simulink model "ndtm_V2"  (R2018b)
settings: configuration reference "Physics" (kept outside this file)
model workspace (MAT data in the model file):
  x0_initialstates = [0 0 0 0 0 0]
undefined symbols (not defined in the file): F0z, h, INIT__initialvalues__Vehicle_InitialPitchRate_radps, INIT__initialvalues__Vehicle_InitialRollRate_radps, INIT__initialvalues__Vehicle_InitialVelocity_mps__1, INIT__initialvalues__Vehicle_InitialVelocity_mps__2, INIT__initialvalues__Vehicle_InitialVelocity_mps__3, INIT__initialvalues__Vehicle_InitialYawRate_radps, SUS__Antisway__c_AntiSwayTSpringFrRe_Nmprad__1, SUS__Antisway__c_AntiSwayTSpringFrRe_Nmprad__2, SUS__Antisway__phi_AntiSwayNeutralAngleFrRe_rad__1, SUS__Antisway__phi_AntiSwayNeutralAngleFrRe_rad__2, SUS__Antisway__r_AntiSwayArmRadiusFrRe_m__1, SUS__Antisway__r_AntiSwayArmRadiusFrRe_m__2, SUS__Compliance__Cz_DamperRateFrRe_Nspm__1, SUS__Compliance__Cz_DamperRateFrRe_Nspm__2, SUS__Compliance__cz_SpringRateFrRe_Npm__1, SUS__Compliance__cz_SpringRateFrRe_Npm__2, SUS__Compliance__F0z_SpringPreloadFrRe_N__1, SUS__Compliance__F0z_SpringPreloadFrRe_N__2, SUS__Compliance__h_InertialFrameOffset_COGtoAxle_m, SUS__Kinematics__k_CamberATSteerCenterF__1, SUS__Kinematics__k_CamberATSteerCenterF__2, SUS__Kinematics__k_CamberVSHeightFrRe__1, SUS__Kinematics__k_CamberVSHeightFrRe__2, SUS__Kinematics__k_CasterATSteerCenterF__1, SUS__Kinematics__k_CasterATSteerCenterF__2, SUS__Kinematics__k_CasterVSHeightFrRe__1, SUS__Kinematics__k_CasterVSHeightFrRe__2, SUS__Kinematics__k_RollSteerVSHeightFrRe_radpm__1, SUS__Kinematics__k_RollSteerVSHeightFrRe_radpm__2, SUS__Kinematics__nu0_ToeATSteerCenterFrRe_rad__1, SUS__Kinematics__nu0_ToeATSteerCenterFrRe_rad__2, tireFL__SCALING__LFZO, tireFR__SCALING__LFZO, tireRL__SCALING__LFZO, tireRR__SCALING__LFZO, VEH, VEH__Aerodynamics__beta_wind_end_rad, VEH__Aerodynamics__beta_wind_start_rad, VEH__Aerodynamics__beta_wind_step_rad, VEH__Aerodynamics__cl_LongitudinalLift, VEH__Aerodynamics__Cs_LatDragCoeff_end, VEH__Aerodynamics__Cs_LatDragCoeff_start, VEH__Aerodynamics__Cs_LatDragCoeff_step, VEH__Aerodynamics__Cym_DragYawMomentCoeff_end, VEH__Aerodynamics__Cym_DragYawMomentCoeff_start, VEH__Aerodynamics__Cym_DragYawMomentCoeff_step, VEH__Environment__a_Gravity_mps2, VEH__Tires__p_Tires_pa__1, VEH__Tires__p_Tires_pa__2, VEH__Tires__p_Tires_pa__3, VEH__Tires__p_Tires_pa__4, VEH__VehicleData__l_WheelbaseF_m, VEH__VehicleData__l_WheelbaseTotal_m, VEH__VehicleData__m_Vehicle_kg, VEH__VehicleData__w_GeomCenterlineToCOG_m, VEH__VehicleData__w_TrackF_m, VEH__VehicleData__w_TrackR_m
libraries: vehdynlibsuspension x7, vehdynlibtire x4, vehdynlibtire_TUM x4, autolibutils x2, sharedtransform x2, vehdynlibeom_TUM x1
(part 4 of 4)

== system ndtm_V2/Wheels and Tires/VDBS/Veh2Tire ==
  r : Inport
  Axle : Inport  Port=2
  Brake : Inport  Port=3
  VehVel : Inport  Port=4
  WheelSteer : Inport  Port=5
  WheelCamber : Inport  Port=6
  Demux4 : Demux
  Gain4 : Gain  Gain=[1;-1;1;-1]*0+1
  Mux1 : Mux
  Reshape3 : Reshape
  Reshape4 : Reshape
  Unary Minus : UnaryMinus
  Wheel Angles : Subsystem
  Wheel to Body Transform : Subsystem
  T : Outport  Unit=N*m
  P : Outport  Port=2  Unit=Pa
  psidot : Outport  Port=3  Unit=rad/s
  xdotAxle : Outport  Port=4  Unit=m/s
  ydotAxle : Outport  Port=5  Unit=m/s
  zdotAxle : Outport  Port=6  Unit=m/s
  wires:
  Demux4/1 -> Mux1/1
  Brake/1 -> Reshape3/1
  Demux4/4 -> Mux1/4
  Axle/1 -> Reshape4/1
  Wheel to Body Transform/1(xdotWheel) -> xdotAxle/1  "Vx"
  Demux4/2 -> Mux1/2
  Wheel to Body Transform/2(ydotWheel) -> ydotAxle/1  "Vy"
  WheelSteer/1 -> Wheel Angles/1(steer)
  Mux1/1 -> P/1
  r/1 -> Unary Minus/1
  Demux4/3 -> Mux1/3
  Reshape3/1 -> Demux4/1
  Gain4/1 -> T/1
  Reshape4/1 -> Gain4/1
  VehVel/1 -> Wheel to Body Transform/1(VelVeh)
  Wheel to Body Transform/3(zdotWheel) -> zdotAxle/1  "Vz"
  WheelCamber/1 -> Wheel Angles/2(camber)
  Unary Minus/1 -> psidot/1
  Wheel Angles/1(Vehicle) -> Wheel to Body Transform/2(WheelAngles)

== system ndtm_V2/Wheels and Tires/VDBS/scale factors with friction ==
  lamda_mu_x : Inport
  lamda_mu_y : Inport  Port=2
  Constant7 : Constant  Value=[tireFL__SCALING__LFZO, tireFR__SCALING__LFZO, tireRL__SCALING__LFZO, tireRR__SCALING__LFZO]
  Reshape : Reshape  OutputDimensionality=Row vector (2-D)  OutputDimensions=[1,numWheels]
  Reshape1 : Reshape  OutputDimensionality=Row vector (2-D)  OutputDimensions=[1,numWheels]
  Reshape6 : Reshape  OutputDimensionality=Row vector (2-D)
  Signal Specification : SignalSpecification  Unit=1
  Signal Specification1 : SignalSpecification  Unit=1
  Vector Concatenate : Concatenate  NumInputs=4  Mode=Multidimensional array
  ones1 : Constant  Value=[ones(24,numWheels)]  VectorParams1D=off
  lambdas : Outport  Unit=1
  wires:
  Reshape1/1 -> Vector Concatenate/3
  Reshape/1 -> Vector Concatenate/2
  lamda_mu_y/1 -> Reshape1/1
  lamda_mu_x/1 -> Reshape/1
  ones1/1 -> Signal Specification1/1
  Reshape6/1 -> Signal Specification/1
  Vector Concatenate/1 -> lambdas/1
  Signal Specification/1 -> Vector Concatenate/1
  Signal Specification1/1 -> Vector Concatenate/4
  Constant7/1 -> Reshape6/1

== system ndtm_V2/Wheels and Tires/VDBS/Tire2Veh/Subsystem ==
  <Mz> : Inport
  <Mx> : Inport  Port=2
  <My> : Inport  Port=3
  <Re> : Inport  Port=4
  <z> : Inport  Port=5
  <zdot> : Inport  Port=6
  <Kappa> : Inport  Port=7
  <Alpha> : Inport  Port=8
  omega : Inport  Port=9
  Fx : Inport  Port=10
  Fy : Inport  Port=11
  Fz : Inport  Port=12
  Bus Creator : BusCreator  Inputs=12
  Reshape : Reshape  OutputDimensionality=Row vector (2-D)
  Reshape1 : Reshape  OutputDimensionality=Row vector (2-D)
  Unary Minus1 : UnaryMinus
  Unary Minus2 : UnaryMinus
  Out1 : Outport
  Out2 : Outport  Port=2
  Out3 : Outport  Port=3
  wires:
  <Re>/1 -> Bus Creator/8
  Unary Minus1/1 -> Reshape/1, Bus Creator/9  "z"
  Fz/1 -> Bus Creator/4
  <zdot>/1 -> Unary Minus2/1
  <Mz>/1 -> Bus Creator/7
  Unary Minus2/1 -> Reshape1/1, Bus Creator/10  "zdot"
  <z>/1 -> Unary Minus1/1
  Bus Creator/1 -> Out1/1
  Fy/1 -> Bus Creator/3
  omega/1 -> Bus Creator/1
  Fx/1 -> Bus Creator/2
  Reshape1/1 -> Out3/1
  <Kappa>/1 -> Bus Creator/11
  Reshape/1 -> Out2/1
  <Mx>/1 -> Bus Creator/5
  <My>/1 -> Bus Creator/6
  <Alpha>/1 -> Bus Creator/12

== system ndtm_V2/Wheels and Tires/VDBS/Tire2Veh/Wheel Angles ==
  Front : Inport
  Camber : Inport  Port=2
  Add1 : Sum
  Add2 : Sum
  Constant1 : Constant  Value=pi
  Constant2 : Constant  Value=[pi;0;pi;0].*0+[0;pi;0;pi].*.0
  Constant3 : Constant  Value=ones(1,4).*0
  Reshape : Reshape  OutputDimensionality=Row vector (2-D)
  Reshape1 : Reshape  OutputDimensionality=Row vector (2-D)
  Reshape2 : Reshape  OutputDimensionality=Row vector (2-D)
  Vector Concatenate3 : Concatenate  NumInputs=3  Mode=Multidimensional array
  Vehicle : Outport
  wires:
  Reshape/1 -> Vector Concatenate3/3
  Reshape2/1 -> Vector Concatenate3/2
  Vector Concatenate3/1 -> Vehicle/1
  Constant2/1 -> Add1/2
  Front/1 -> Add1/1
  Reshape1/1 -> Vector Concatenate3/1
  Constant3/1 -> Reshape2/1
  Add1/1 -> Reshape/1
  Camber/1 -> Add2/1
  Add2/1 -> Reshape1/1
  Constant1/1 -> Add2/2

== system ndtm_V2/Wheels and Tires/VDBS/Tire2Veh/Wheel to Body Transform ==
  Forces : Inport  Partition=on  PartitionDimension=2  PartitionWidth=1  PartitionOffset=0
  WheelAngles : Inport  Port=2  Partition=on  PartitionDimension=2  PartitionWidth=1  PartitionOffset=0
  Demux1 : Demux  Outputs=3
  Divide1 : Product  Inputs=**  Multiplication=Matrix(*)
  For Each : ForEach  DisableCoverage=on  IndexMode=One-based
  Rotation Angles to Direction Cosine Matrix : sharedtransform/Rotation Angles to Direction Cosine Matrix  rotationOrder=ZYX  aMode=2
      settings: SourceProductBaseCode=AE
  Selector : Selector  InputPortWidth=3  IndexOptions=Index vector (dialog)  Indices=[3 2 1]  OutputSizes=1
  Fx : Outport  ConcatenationDimension=1
  Fy : Outport  Port=2  ConcatenationDimension=1
  Fz : Outport  Port=3  ConcatenationDimension=1
  wires:
  Divide1/1 -> Demux1/1
  Demux1/1 -> Fx/1
  Demux1/2 -> Fy/1
  Demux1/3 -> Fz/1
  Rotation Angles to Direction Cosine Matrix/1 -> Divide1/1
  Forces/1 -> Divide1/2
  WheelAngles/1 -> Selector/1
  Selector/1 -> Rotation Angles to Direction Cosine Matrix/1

== system ndtm_V2/Wheels and Tires/VDBS/Tires/Fx ==
  In1 : Inport
  In2 : Inport  Port=2
  In3 : Inport  Port=3
  In4 : Inport  Port=4
  Bus Selector{,1..3} (4 alike) : BusSelector  OutputSignals=Fx
  Vector Concatenate : Concatenate  NumInputs=4
  Out1 : Outport
  wires:
  Bus Selector3/1 -> Vector Concatenate/4  "<Fx>"
  Bus Selector2/1 -> Vector Concatenate/3  "<Fx>"
  Bus Selector1/1 -> Vector Concatenate/2  "<Fx>"
  In4/1 -> Bus Selector3/1
  In3/1 -> Bus Selector2/1
  In2/1 -> Bus Selector1/1
  Bus Selector/1 -> Vector Concatenate/1  "<Fx>"
  In1/1 -> Bus Selector/1
  Vector Concatenate/1 -> Out1/1

== system ndtm_V2/Wheels and Tires/VDBS/Tires/Fy ==
  In1 : Inport
  In2 : Inport  Port=2
  In3 : Inport  Port=3
  In4 : Inport  Port=4
  Bus Selector{,1..3} (4 alike) : BusSelector  OutputSignals=Fy
  Vector Concatenate : Concatenate  NumInputs=4
  Out1 : Outport
  wires:
  Vector Concatenate/1 -> Out1/1
  In1/1 -> Bus Selector/1
  Bus Selector/1 -> Vector Concatenate/1  "<Fy>"
  In2/1 -> Bus Selector1/1
  In3/1 -> Bus Selector2/1
  In4/1 -> Bus Selector3/1
  Bus Selector1/1 -> Vector Concatenate/2  "<Fy>"
  Bus Selector2/1 -> Vector Concatenate/3  "<Fy>"
  Bus Selector3/1 -> Vector Concatenate/4  "<Fy>"

== system ndtm_V2/Wheels and Tires/VDBS/Tires/Fz ==
  In1 : Inport
  In2 : Inport  Port=2
  In3 : Inport  Port=3
  In4 : Inport  Port=4
  Bus Selector{,1..3} (4 alike) : BusSelector  OutputSignals=Fz
  Vector Concatenate : Concatenate  NumInputs=4
  Out1 : Outport
  wires:
  Vector Concatenate/1 -> Out1/1
  In1/1 -> Bus Selector/1
  Bus Selector/1 -> Vector Concatenate/1  "<Fz>"
  In2/1 -> Bus Selector1/1
  In3/1 -> Bus Selector2/1
  In4/1 -> Bus Selector3/1
  Bus Selector1/1 -> Vector Concatenate/2  "<Fz>"
  Bus Selector2/1 -> Vector Concatenate/3  "<Fz>"
  Bus Selector3/1 -> Vector Concatenate/4  "<Fz>"

== system ndtm_V2/Wheels and Tires/VDBS/Tires/Mx ==
  In1 : Inport
  In2 : Inport  Port=2
  In3 : Inport  Port=3
  In4 : Inport  Port=4
  Bus Selector{,1..3} (4 alike) : BusSelector  OutputSignals=Mx
  Vector Concatenate : Concatenate  NumInputs=4
  Out1 : Outport
  wires:
  Vector Concatenate/1 -> Out1/1
  In1/1 -> Bus Selector/1
  Bus Selector/1 -> Vector Concatenate/1  "<Mx>"
  In2/1 -> Bus Selector1/1
  In3/1 -> Bus Selector2/1
  In4/1 -> Bus Selector3/1
  Bus Selector1/1 -> Vector Concatenate/2  "<Mx>"
  Bus Selector2/1 -> Vector Concatenate/3  "<Mx>"
  Bus Selector3/1 -> Vector Concatenate/4  "<Mx>"

== system ndtm_V2/Wheels and Tires/VDBS/Tires/My ==
  In1 : Inport
  In2 : Inport  Port=2
  In3 : Inport  Port=3
  In4 : Inport  Port=4
  Bus Selector{,1..3} (4 alike) : BusSelector  OutputSignals=My
  Vector Concatenate : Concatenate  NumInputs=4
  Out1 : Outport
  wires:
  Bus Selector3/1 -> Vector Concatenate/4  "<My>"
  Bus Selector2/1 -> Vector Concatenate/3  "<My>"
  Bus Selector1/1 -> Vector Concatenate/2  "<My>"
  In4/1 -> Bus Selector3/1
  In3/1 -> Bus Selector2/1
  In2/1 -> Bus Selector1/1
  Bus Selector/1 -> Vector Concatenate/1  "<My>"
  In1/1 -> Bus Selector/1
  Vector Concatenate/1 -> Out1/1

== system ndtm_V2/Wheels and Tires/VDBS/Tires/Mz ==
  In1 : Inport
  In2 : Inport  Port=2
  In3 : Inport  Port=3
  In4 : Inport  Port=4
  Bus Selector{,1..3} (4 alike) : BusSelector  OutputSignals=Mz
  Vector Concatenate : Concatenate  NumInputs=4
  Out1 : Outport
  wires:
  Bus Selector3/1 -> Vector Concatenate/4  "<Mz>"
  Bus Selector2/1 -> Vector Concatenate/3  "<Mz>"
  Bus Selector1/1 -> Vector Concatenate/2  "<Mz>"
  In4/1 -> Bus Selector3/1
  In3/1 -> Bus Selector2/1
  In2/1 -> Bus Selector1/1
  Bus Selector/1 -> Vector Concatenate/1  "<Mz>"
  In1/1 -> Bus Selector/1
  Vector Concatenate/1 -> Out1/1

== system ndtm_V2/Wheels and Tires/VDBS/Tires/Re ==
  In1 : Inport
  In2 : Inport  Port=2
  In3 : Inport  Port=3
  In4 : Inport  Port=4
  Bus Selector{,1..3} (4 alike) : BusSelector  OutputSignals=Re
  Vector Concatenate : Concatenate  NumInputs=4
  Out1 : Outport
  wires:
  Vector Concatenate/1 -> Out1/1
  In1/1 -> Bus Selector/1
  Bus Selector/1 -> Vector Concatenate/1  "<Re>"
  In2/1 -> Bus Selector1/1
  In3/1 -> Bus Selector2/1
  In4/1 -> Bus Selector3/1
  Bus Selector1/1 -> Vector Concatenate/2  "<Re>"
  Bus Selector2/1 -> Vector Concatenate/3  "<Re>"
  Bus Selector3/1 -> Vector Concatenate/4  "<Re>"

== system ndtm_V2/Wheels and Tires/VDBS/Tires/alpha ==
  In1 : Inport
  In2 : Inport  Port=2
  In3 : Inport  Port=3
  In4 : Inport  Port=4
  Bus Selector{,1..3} (4 alike) : BusSelector  OutputSignals=Alpha
  Vector Concatenate : Concatenate  NumInputs=4
  Out1 : Outport
  wires:
  Vector Concatenate/1 -> Out1/1
  In1/1 -> Bus Selector/1
  Bus Selector/1 -> Vector Concatenate/1  "<Alpha>"
  In2/1 -> Bus Selector1/1
  In3/1 -> Bus Selector2/1
  In4/1 -> Bus Selector3/1
  Bus Selector1/1 -> Vector Concatenate/2  "<Alpha>"
  Bus Selector2/1 -> Vector Concatenate/3  "<Alpha>"
  Bus Selector3/1 -> Vector Concatenate/4  "<Alpha>"

== system ndtm_V2/Wheels and Tires/VDBS/Tires/kappa ==
  In1 : Inport
  In2 : Inport  Port=2
  In3 : Inport  Port=3
  In4 : Inport  Port=4
  Bus Selector{,1..3} (4 alike) : BusSelector  OutputSignals=Kappa
  Vector Concatenate : Concatenate  NumInputs=4
  Out1 : Outport
  wires:
  Bus Selector3/1 -> Vector Concatenate/4  "<Kappa>"
  Bus Selector2/1 -> Vector Concatenate/3  "<Kappa>"
  Bus Selector1/1 -> Vector Concatenate/2  "<Kappa>"
  In4/1 -> Bus Selector3/1
  In3/1 -> Bus Selector2/1
  In2/1 -> Bus Selector1/1
  Bus Selector/1 -> Vector Concatenate/1  "<Kappa>"
  In1/1 -> Bus Selector/1
  Vector Concatenate/1 -> Out1/1

== system ndtm_V2/Wheels and Tires/VDBS/Tires/omega ==
  In1 : Inport
  In2 : Inport  Port=2
  In3 : Inport  Port=3
  In4 : Inport  Port=4
  Bus Selector{,1..3} (4 alike) : BusSelector  OutputSignals=Omega
  Vector Concatenate : Concatenate  NumInputs=4
  Out1 : Outport
  wires:
  In1/1 -> Bus Selector/1
  Bus Selector/1 -> Vector Concatenate/1  "<Omega>"
  In2/1 -> Bus Selector1/1
  In3/1 -> Bus Selector2/1
  In4/1 -> Bus Selector3/1
  Bus Selector1/1 -> Vector Concatenate/2  "<Omega>"
  Bus Selector2/1 -> Vector Concatenate/3  "<Omega>"
  Bus Selector3/1 -> Vector Concatenate/4  "<Omega>"
  Vector Concatenate/1 -> Out1/1

== system ndtm_V2/Wheels and Tires/VDBS/Tires/z ==
  In1 : Inport
  In2 : Inport  Port=2
  In3 : Inport  Port=3
  In4 : Inport  Port=4
  Bus Selector{,1..3} (4 alike) : BusSelector  OutputSignals=z
  Vector Concatenate : Concatenate  NumInputs=4
  Out1 : Outport
  wires:
  Bus Selector3/1 -> Vector Concatenate/4  "<z>"
  Bus Selector2/1 -> Vector Concatenate/3  "<z>"
  Bus Selector1/1 -> Vector Concatenate/2  "<z>"
  In4/1 -> Bus Selector3/1
  In3/1 -> Bus Selector2/1
  In2/1 -> Bus Selector1/1
  Bus Selector/1 -> Vector Concatenate/1  "<z>"
  In1/1 -> Bus Selector/1
  Vector Concatenate/1 -> Out1/1

== system ndtm_V2/Wheels and Tires/VDBS/Tires/zdot ==
  In1 : Inport
  In2 : Inport  Port=2
  In3 : Inport  Port=3
  In4 : Inport  Port=4
  Bus Selector{,1..3} (4 alike) : BusSelector  OutputSignals=zdot
  Vector Concatenate : Concatenate  NumInputs=4
  Out1 : Outport
  wires:
  Vector Concatenate/1 -> Out1/1
  In1/1 -> Bus Selector/1
  Bus Selector/1 -> Vector Concatenate/1  "<zdot>"
  In2/1 -> Bus Selector1/1
  In3/1 -> Bus Selector2/1
  In4/1 -> Bus Selector3/1
  Bus Selector1/1 -> Vector Concatenate/2  "<zdot>"
  Bus Selector2/1 -> Vector Concatenate/3  "<zdot>"
  Bus Selector3/1 -> Vector Concatenate/4  "<zdot>"

== system ndtm_V2/Wheels and Tires/VDBS/Veh2Tire/Wheel Angles ==
  steer : Inport
  camber : Inport  Port=2
  Add1 : Sum
  Add2 : Sum
  Constant1 : Constant  Value=pi
  Constant2 : Constant  Value=[pi;0;pi;0].*0+[0;pi;0;pi].*0
  Constant3 : Constant  Value=ones(1,4).*0
  Reshape : Reshape  OutputDimensionality=Row vector (2-D)
  Reshape1 : Reshape  OutputDimensionality=Row vector (2-D)
  Reshape2 : Reshape  OutputDimensionality=Row vector (2-D)
  Vector Concatenate3 : Concatenate  NumInputs=3  Mode=Multidimensional array
  Vehicle : Outport
  wires:
  Constant2/1 -> Add1/2
  Constant3/1 -> Reshape2/1
  Vector Concatenate3/1 -> Vehicle/1
  Reshape/1 -> Vector Concatenate3/3
  Reshape1/1 -> Vector Concatenate3/1
  camber/1 -> Add2/1
  Reshape2/1 -> Vector Concatenate3/2
  steer/1 -> Add1/1
  Add1/1 -> Reshape/1
  Constant1/1 -> Add2/2
  Add2/1 -> Reshape1/1

== system ndtm_V2/Wheels and Tires/VDBS/Veh2Tire/Wheel to Body Transform ==
  VelVeh : Inport  Partition=on  PartitionDimension=2  PartitionWidth=1  PartitionOffset=0
  WheelAngles : Inport  Port=2  Partition=on  PartitionDimension=2  PartitionWidth=1  PartitionOffset=0
  Demux1 : Demux  Outputs=3
  Divide1 : Product  Inputs=**  Multiplication=Matrix(*)
  For Each : ForEach  DisableCoverage=on  IndexMode=One-based
  Rotation Angles to Direction Cosine Matrix : sharedtransform/Rotation Angles to Direction Cosine Matrix  rotationOrder=ZYX  aMode=2
      settings: SourceProductBaseCode=AE
  Selector : Selector  InputPortWidth=3  IndexOptions=Index vector (dialog)  Indices=[3 2 1]  OutputSizes=1
  xdotWheel : Outport  ConcatenationDimension=1
  ydotWheel : Outport  Port=2  ConcatenationDimension=1
  zdotWheel : Outport  Port=3  ConcatenationDimension=1
  wires:
  Divide1/1 -> Demux1/1
  Demux1/1 -> xdotWheel/1
  Demux1/2 -> ydotWheel/1
  Demux1/3 -> zdotWheel/1
  Rotation Angles to Direction Cosine Matrix/1 -> Divide1/1
  VelVeh/1 -> Divide1/2
  WheelAngles/1 -> Selector/1
  Selector/1 -> Rotation Angles to Direction Cosine Matrix/1
